simulink model "systemOffLine"  (Simulink 8.5)
settings: Solver=ode3  SolverMode=SingleTasking  StartTime=0.0  StopTime=0.1  RelTol=1e-3  AbsTol=1e-6
undefined symbols (not defined in the file or in its folder): DAB, den, elements, num
(part 1 of 5)
settings Model: Creator=PC  LastModifiedBy=PC  ExtModeTrigMode=oneshot  ExtModeArmWhenConnect=off
settings DataIOCC: LimitDataPoints=off
settings OptimizationCC: BlockReduction=off  BooleanDataType=off  ExpressionDepthLimit=128
settings DebuggingCC: SaveWithParameterizedLinksMsg=none  SignalResolutionControl=TryResolveAllWithWarning  MultiTaskDSMMsg=warning  MultiTaskCondExecSysMsg=none  FcnCallInpInsideContextMsg=EnableAllAsError  StateNameClashWarn=none
settings HardwareCC: TargetUnknown=on

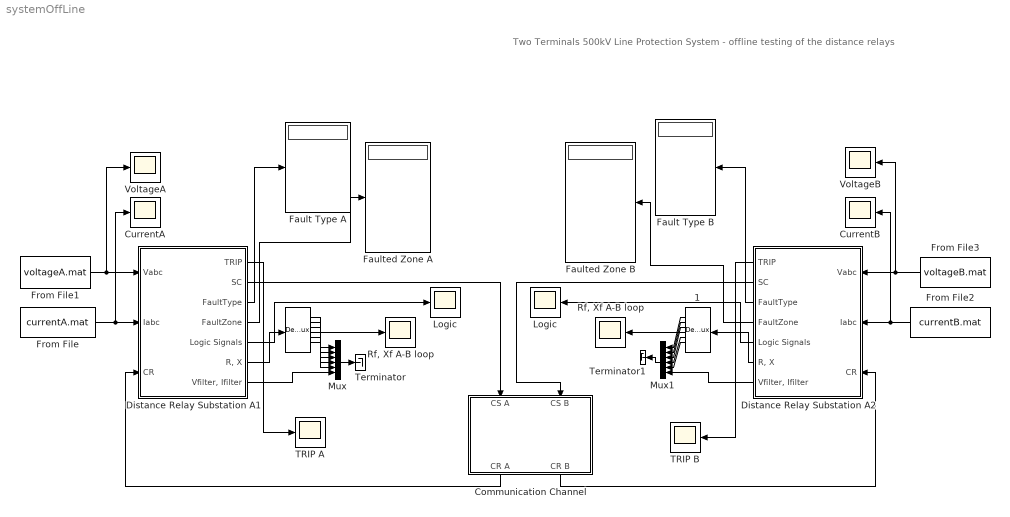
== system systemOffLine ==
  note: Two Terminals 500kV Line Protection System - offline testing of the distance relays
  "    " : Demux  Outputs=6
  "    1" : Demux  Outputs=6
  Communication Channel : Subsystem  mask(Communication channel.){Tdelay=20, failure=off, err_signal=0}
      mask prompts: Tdelay "Channel delay time [ms]:"; failure "Communication channel failure."; err_signal "Erroneous signal:"
      mask TypeOptions err_signal: 0 | 1
  CurrentA : Scope
      settings: TickLabels=on
  CurrentB : Scope
      settings: TickLabels=on
  Distance Relay Substation A1 : Subsystem  mask{ZoneImpedance=[90 115 200 250 50], ZoneTime=[0 0.33 1 0.33 0.66], k0m1=0.726, k0a1=-3.69, LineAngle=84, Zstarter=300, Tstarter=0, underV=0.8*500000/sqrt(3)*sqrt(2), PilotLogic='PUTT', fCut=180, fSampling=24*60, WindowSize=24, VoltageRange=480, CurrentRange=480}
      mask prompts: ZoneImpedance "Zone Impedances [Z1 Z2 Z3 Z4 ZR] (Ohm):"; ZoneTime "Zone Times [T1 T2 T3 T4 TR] (s):"; LineAngle "Line Angle:"; Zstarter "Starter Impedance (Ohm):"; Tstarter "Starter Time (s):"; underV "UnderVoltage Threshold (V):"; PilotLogic "Pilot Logic Scheme:"; fCut "fCut (Hz):"; fSampling "fSampling (Hz):"; WindowSize "Window Size (samples):"; VoltageRange "Voltage Range (V):"; CurrentRange "Current Range (A):"
      mask TypeOptions PilotLogic: 'BLOV+TB' | 'PUTT'
  Distance Relay Substation A2 : Subsystem  mask{ZoneImpedance=[90 115 200 250 50], ZoneTime=[0 0.33 1 0.33 0.66], k0m1=0.726, k0a1=-3.69, LineAngle=84, Zstarter=300, Tstarter=0, underV=0.8*1.05*500000/sqrt(3)*sqrt(2), PilotLogic='PUTT', fCut=180, fSampling=24*60, WindowSize=24, VoltageRange=480, CurrentRange=480}
      mask prompts: ZoneImpedance "Zone Impedances [Z1 Z2 Z3 Z4 ZR] (Ohm):"; ZoneTime "Zone Times [T1 T2 T3 T4 TR] (s):"; LineAngle "Line Angle:"; Zstarter "Starter Impedance (Ohm):"; Tstarter "Starter Time (s):"; underV "UnderVoltage Threshold (V):"; PilotLogic "Pilot Logic Scheme:"; fCut "fCut (Hz):"; fSampling "fSampling (Hz):"; WindowSize "Window Size (samples):"; VoltageRange "Voltage Range (V):"; CurrentRange "Current Range (A):"
      mask TypeOptions PilotLogic: 'BLOV+TB' | 'PUTT'
  Fault Type A : Display
  Fault Type B : Display
  Faulted Zone A : Display
  Faulted Zone B : Display
  From File : FromFile  FileName=currentA.mat  SampleTime=0
  From File1 : FromFile  FileName=voltageA.mat  SampleTime=0
  From File2 : FromFile  FileName=currentB.mat  SampleTime=0
  From File3 : FromFile  FileName=voltageB.mat  SampleTime=0
  Logic : Scope
      settings: TickLabels=on  YMin=0  YMax=1
  "Logic " : Scope
      settings: TickLabels=on  YMin=-0.5  YMax=6.5
  Mux : Mux  Inputs=6
  Mux1 : Mux  Inputs=6
  "Rf, Xf A-B loop" : Scope
      settings: TickLabels=on  YMin=-1000  YMax=2250
  "Rf, Xf A-B loop " : Scope
      settings: TickLabels=on  YMin=-150  YMax=700
  TRIP A : Scope
      settings: TickLabels=on  YMin=-1  YMax=1
  TRIP B : Scope
      settings: TickLabels=on  YMin=-1  YMax=1
  Terminator : Terminator
  Terminator1 : Terminator
  VoltageA : Scope
      settings: TickLabels=on  YMin=-450000  YMax=450000
  VoltageB : Scope
      settings: TickLabels=on  YMin=-450000  YMax=450000
  wires:
  "    1"/4 -> "Rf, Xf A-B loop "/1
  "    "/4 -> "Rf, Xf A-B loop"/1
  From File/1 -> Distance Relay Substation A1/2(Iabc), CurrentA/1
  From File1/1 -> VoltageA/1, Distance Relay Substation A1/1(Vabc)
  From File2/1 -> Distance Relay Substation A2/2(Iabc), CurrentB/1
  From File3/1 -> Distance Relay Substation A2/1(Vabc), VoltageB/1
  "    "/1 -> Mux/1
  "    "/2 -> Mux/2
  "    "/3 -> Mux/3
  "    "/5 -> Mux/4
  "    "/6 -> Mux/5
  "    1"/1 -> Mux1/1
  "    1"/2 -> Mux1/2
  "    1"/3 -> Mux1/3
  "    1"/6 -> Mux1/5
  "    1"/5 -> Mux1/4
  Mux/1 -> Terminator/1
  Mux1/1 -> Terminator1/1
  Communication Channel/1(CR A) -> Distance Relay Substation A1/3(CR)
  Distance Relay Substation A1/1("TRIP ") -> TRIP A/1
  Distance Relay Substation A1/2(SC) -> Communication Channel/1(CS A)
  Distance Relay Substation A1/3(FaultType) -> Fault Type A/1
  Distance Relay Substation A1/4(FaultZone) -> Faulted Zone A/1
  Distance Relay Substation A1/5(Logic Signals) -> Logic/1
  Distance Relay Substation A1/6("R, X") -> "    "/1
  Distance Relay Substation A1/7("Vfilter, Ifilter") -> Mux/6
  Communication Channel/2(CR B) -> Distance Relay Substation A2/3(CR)
  Distance Relay Substation A2/1("TRIP ") -> TRIP B/1
  Distance Relay Substation A2/2(SC) -> Communication Channel/2(CS B)
  Distance Relay Substation A2/3(FaultType) -> Fault Type B/1
  Distance Relay Substation A2/4(FaultZone) -> Faulted Zone B/1
  Distance Relay Substation A2/5(Logic Signals) -> "Logic "/1
  Distance Relay Substation A2/6("R, X") -> "    1"/1
  Distance Relay Substation A2/7("Vfilter, Ifilter") -> Mux1/6

== system systemOffLine/Communication Channel ==
  CS A : Inport
  CS B : Inport  Port=2
  " " : Constant  Value=failure
  "  " : Constant  Value=err_signal-1
  Switch : Switch  Threshold=0.5  SaturateOnIntegerOverflow=on  InputSameDT=on
  Switch1 : Switch  Threshold=0.5  SaturateOnIntegerOverflow=on  InputSameDT=on
  delay A->B : TransportDelay  DelayTime=Tdelay/1000  BufferSize=2048
  delay B->A : TransportDelay  DelayTime=Tdelay/1000  BufferSize=2048
  CR A : Outport  InitialOutput=0
  CR B : Outport  Port=2  InitialOutput=0
  wires:
  " "/1 -> Switch1/2, Switch/2
  delay B->A/1 -> Switch1/3
  delay A->B/1 -> Switch/3
  "  "/1 -> Switch/1, Switch1/1
  Switch1/1 -> CR B/1
  CS A/1 -> delay B->A/1
  CS B/1 -> delay A->B/1
  Switch/1 -> CR A/1

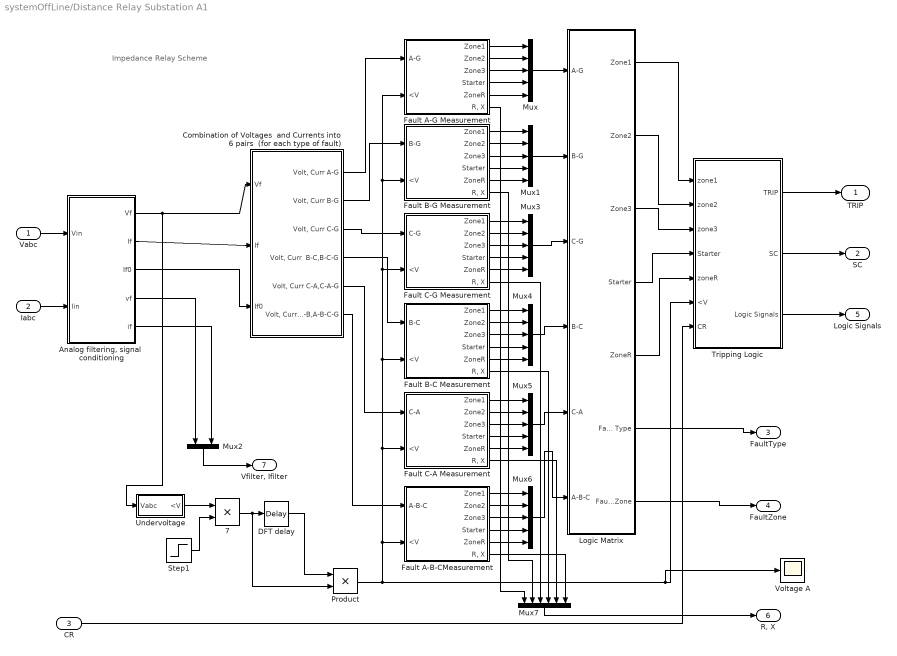
== system systemOffLine/Distance Relay Substation A1 ==
  note: Impedance Relay Scheme
  Vabc : Inport
  Iabc : Inport  Port=2
  CR : Inport  Port=3
  " 7" : Product  RndMeth=Zero
  "Analog filtering, signal  conditioning" : Subsystem
  Combination of Voltages  and Currents into 6 pairs  (for each type of fault) : Subsystem
  DFT delay : TransportDelay  DelayTime=0.017  BufferSize=30720
  Fault A-B-CMeasurement : Subsystem
  Fault A-G Measurement : Subsystem
  Fault B-C Measurement : Subsystem
  Fault B-G Measurement : Subsystem
  Fault C-A Measurement : Subsystem
  Fault C-G Measurement : Subsystem
  Logic Matrix : Subsystem
  Mux{,1,3..6} (6 alike) : Mux  Inputs=5
  Mux2 : Mux  Inputs=2
  Mux7 : Mux  Inputs=6
  Product : Product  RndMeth=Zero
  Step1 : Step  Time=0.017  SampleTime=0
  Tripping Logic : Subsystem
  Undervoltage : Subsystem
  Voltage A : Scope
      settings: TickLabels=on  YMin=-400000  YMax=400000  SaveName=ScopeData9
  "TRIP " : Outport  InitialOutput=0
  SC : Outport  Port=2  InitialOutput=0
  FaultType : Outport  Port=3  InitialOutput=0
  FaultZone : Outport  Port=4  InitialOutput=0
  Logic Signals : Outport  Port=5  InitialOutput=0
  "R, X" : Outport  Port=6  InitialOutput=0
  "Vfilter, Ifilter" : Outport  Port=7  InitialOutput=0
  wires:
  Mux2/1 -> "Vfilter, Ifilter"/1
  Product/1 -> Fault A-B-CMeasurement/2(<V), Fault C-A Measurement/2(<V), Fault B-C Measurement/2(<V), Fault C-G Measurement/2(<V), Fault B-G Measurement/2(<V), Fault A-G Measurement/2(<V), Voltage A/1, Tripping Logic/6(<V)
  Logic Matrix/6(Fault Type) -> FaultType/1
  Tripping Logic/1(TRIP) -> "TRIP "/1
  Logic Matrix/3(" Zone3") -> Tripping Logic/3(zone3)
  Logic Matrix/2(" Zone2") -> Tripping Logic/2(zone2)
  Logic Matrix/1(" Zone1") -> Tripping Logic/1(zone1)
  Mux6/1 -> Logic Matrix/6(A-B-C)
  Mux5/1 -> Logic Matrix/5(C-A)
  Mux4/1 -> Logic Matrix/4(B-C)
  Mux3/1 -> Logic Matrix/3(C-G)
  Mux1/1 -> Logic Matrix/2(B-G)
  Mux/1 -> Logic Matrix/1(A-G)
  Fault B-G Measurement/2(Zone2) -> Mux1/2
  Fault A-G Measurement/4(Starter) -> Mux/4
  Fault A-G Measurement/3(Zone3) -> Mux/3
  Fault A-G Measurement/2(Zone2) -> Mux/2
  Fault A-G Measurement/1(Zone1) -> Mux/1
  DFT delay/1 -> Product/1
  Combination of Voltages  and Currents into 6 pairs  (for each type of fault)/5("Volt, Curr C-A,C-A-G") -> Fault C-A Measurement/1(C-A)
  Combination of Voltages  and Currents into 6 pairs  (for each type of fault)/2("Volt, Curr B-G") -> Fault B-G Measurement/1(B-G)
  "Analog filtering, signal  conditioning"/3(If0) -> Combination of Voltages  and Currents into 6 pairs  (for each type of fault)/3(If0)
  "Analog filtering, signal  conditioning"/2(If) -> Combination of Voltages  and Currents into 6 pairs  (for each type of fault)/2(If)
  "Analog filtering, signal  conditioning"/5(if) -> Mux2/2
  "Analog filtering, signal  conditioning"/4(vf) -> Mux2/1
  "Analog filtering, signal  conditioning"/1(Vf) -> Undervoltage/1("Vabc  "), Combination of Voltages  and Currents into 6 pairs  (for each type of fault)/1(Vf)
  " 7"/1 -> Product/2, DFT delay/1
  Step1/1 -> " 7"/2
  Undervoltage/1(<V) -> " 7"/1
  Combination of Voltages  and Currents into 6 pairs  (for each type of fault)/1("Volt, Curr A-G") -> Fault A-G Measurement/1(A-G)
  Iabc/1 -> "Analog filtering, signal  conditioning"/2(Iin)
  Vabc/1 -> "Analog filtering, signal  conditioning"/1(Vin)
  Fault B-G Measurement/1(Zone1) -> Mux1/1
  Fault B-G Measurement/3(Zone3) -> Mux1/3
  Fault A-G Measurement/5(ZoneR) -> Mux/5
  Fault B-G Measurement/4(Starter) -> Mux1/4
  Fault B-G Measurement/5(ZoneR) -> Mux1/5
  Combination of Voltages  and Currents into 6 pairs  (for each type of fault)/3("Volt, Curr C-G") -> Fault C-G Measurement/1(C-G)
  Fault C-G Measurement/1(Zone1) -> Mux3/1
  Fault C-G Measurement/2(Zone2) -> Mux3/2
  Fault C-G Measurement/3(Zone3) -> Mux3/3
  Fault C-G Measurement/4(Starter) -> Mux3/4
  Fault C-G Measurement/5(ZoneR) -> Mux3/5
  Combination of Voltages  and Currents into 6 pairs  (for each type of fault)/4("Volt, Curr  B-C,B-C-G") -> Fault B-C Measurement/1(B-C)
  Fault B-C Measurement/1(Zone1) -> Mux4/1
  Fault B-C Measurement/2(Zone2) -> Mux4/2
  Fault B-C Measurement/3(Zone3) -> Mux4/3
  Fault B-C Measurement/4(Starter) -> Mux4/4
  Fault B-C Measurement/5(ZoneR) -> Mux4/5
  Fault C-A Measurement/1(Zone1) -> Mux5/1
  Fault C-A Measurement/2(Zone2) -> Mux5/2
  Fault C-A Measurement/3(Zone3) -> Mux5/3
  Fault C-A Measurement/4(Starter) -> Mux5/4
  Fault C-A Measurement/5(ZoneR) -> Mux5/5
  Fault A-B-CMeasurement/1(Zone1) -> Mux6/1
  Fault A-B-CMeasurement/2(Zone2) -> Mux6/2
  Fault A-B-CMeasurement/3(Zone3) -> Mux6/3
  Fault A-B-CMeasurement/4(Starter) -> Mux6/4
  Fault A-B-CMeasurement/5(ZoneR) -> Mux6/5
  Combination of Voltages  and Currents into 6 pairs  (for each type of fault)/6("Volt, Curr A-B,A-B-C-G") -> Fault A-B-CMeasurement/1(A-B-C)
  Mux7/1 -> "R, X"/1
  Fault A-B-CMeasurement/6("R, X") -> Mux7/6
  Fault C-A Measurement/6("R, X") -> Mux7/5
  Fault B-C Measurement/6("R, X") -> Mux7/4
  Fault C-G Measurement/6("R, X") -> Mux7/3
  Fault B-G Measurement/6("R, X") -> Mux7/2
  Fault A-G Measurement/6("R, X") -> Mux7/1
  Logic Matrix/7(Fault Zone) -> FaultZone/1
  Tripping Logic/2(SC) -> SC/1
  Tripping Logic/3(Logic Signals) -> Logic Signals/1
  CR/1 -> Tripping Logic/7(CR)
  Logic Matrix/4(" Starter") -> Tripping Logic/4(Starter)
  Logic Matrix/5(" ZoneR") -> Tripping Logic/5(zoneR)

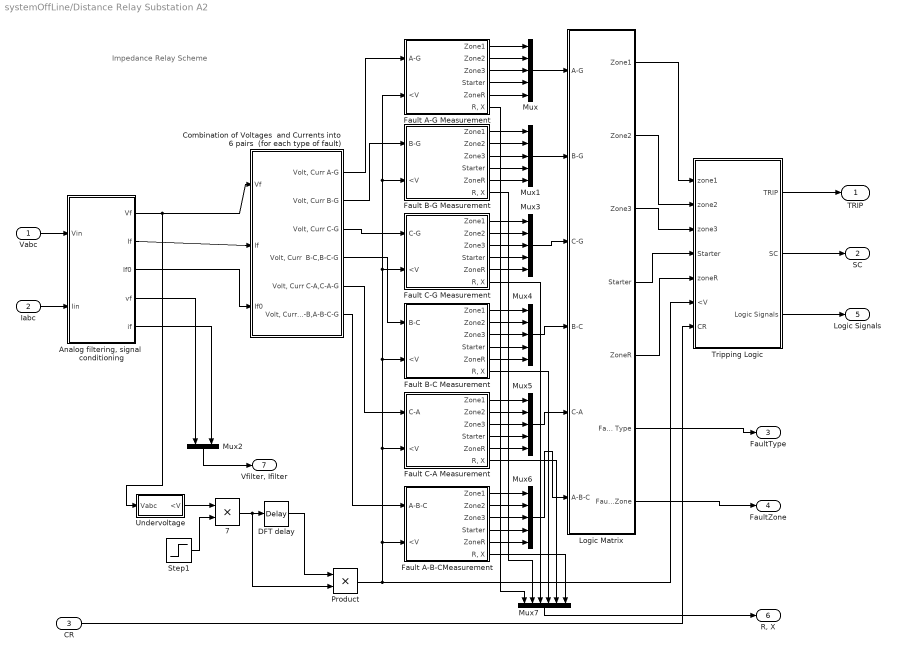
== system systemOffLine/Distance Relay Substation A2 ==
  note: Impedance Relay Scheme
  Vabc : Inport
  Iabc : Inport  Port=2
  CR : Inport  Port=3
  " 7" : Product  RndMeth=Zero
  "Analog filtering, signal  conditioning" : Subsystem
  Combination of Voltages  and Currents into 6 pairs  (for each type of fault) : Subsystem
  DFT delay : TransportDelay  DelayTime=0.017  BufferSize=30720
  Fault A-B-CMeasurement : Subsystem
  Fault A-G Measurement : Subsystem
  Fault B-C Measurement : Subsystem
  Fault B-G Measurement : Subsystem
  Fault C-A Measurement : Subsystem
  Fault C-G Measurement : Subsystem
  Logic Matrix : Subsystem
  Mux{,1,3..6} (6 alike) : Mux  Inputs=5
  Mux2 : Mux  Inputs=2
  Mux7 : Mux  Inputs=6
  Product : Product  RndMeth=Zero
  Step1 : Step  Time=0.017  SampleTime=0
  Tripping Logic : Subsystem
  Undervoltage : Subsystem
  "TRIP " : Outport  InitialOutput=0
  SC : Outport  Port=2  InitialOutput=0
  FaultType : Outport  Port=3  InitialOutput=0
  FaultZone : Outport  Port=4  InitialOutput=0
  Logic Signals : Outport  Port=5  InitialOutput=0
  "R, X" : Outport  Port=6  InitialOutput=0
  "Vfilter, Ifilter" : Outport  Port=7  InitialOutput=0
  wires:
  Mux2/1 -> "Vfilter, Ifilter"/1
  Product/1 -> Fault A-B-CMeasurement/2(<V), Fault C-A Measurement/2(<V), Fault B-C Measurement/2(<V), Fault C-G Measurement/2(<V), Fault B-G Measurement/2(<V), Fault A-G Measurement/2(<V), Tripping Logic/6(<V)
  Logic Matrix/6(Fault Type) -> FaultType/1
  Tripping Logic/1(TRIP) -> "TRIP "/1
  Logic Matrix/3(" Zone3") -> Tripping Logic/3(zone3)
  Logic Matrix/2(" Zone2") -> Tripping Logic/2(zone2)
  Logic Matrix/1(" Zone1") -> Tripping Logic/1(zone1)
  Mux6/1 -> Logic Matrix/6(A-B-C)
  Mux5/1 -> Logic Matrix/5(C-A)
  Mux4/1 -> Logic Matrix/4(B-C)
  Mux3/1 -> Logic Matrix/3(C-G)
  Mux1/1 -> Logic Matrix/2(B-G)
  Mux/1 -> Logic Matrix/1(A-G)
  Fault B-G Measurement/2(Zone2) -> Mux1/2
  Fault A-G Measurement/4(Starter) -> Mux/4
  Fault A-G Measurement/3(Zone3) -> Mux/3
  Fault A-G Measurement/2(Zone2) -> Mux/2
  Fault A-G Measurement/1(Zone1) -> Mux/1
  DFT delay/1 -> Product/1
  Combination of Voltages  and Currents into 6 pairs  (for each type of fault)/5("Volt, Curr C-A,C-A-G") -> Fault C-A Measurement/1(C-A)
  Combination of Voltages  and Currents into 6 pairs  (for each type of fault)/2("Volt, Curr B-G") -> Fault B-G Measurement/1(B-G)
  "Analog filtering, signal  conditioning"/3(If0) -> Combination of Voltages  and Currents into 6 pairs  (for each type of fault)/3(If0)
  "Analog filtering, signal  conditioning"/2(If) -> Combination of Voltages  and Currents into 6 pairs  (for each type of fault)/2(If)
  "Analog filtering, signal  conditioning"/5(if) -> Mux2/2
  "Analog filtering, signal  conditioning"/4(vf) -> Mux2/1
  "Analog filtering, signal  conditioning"/1(Vf) -> Undervoltage/1("Vabc  "), Combination of Voltages  and Currents into 6 pairs  (for each type of fault)/1(Vf)
  " 7"/1 -> Product/2, DFT delay/1
  Step1/1 -> " 7"/2
  Undervoltage/1(<V) -> " 7"/1
  Combination of Voltages  and Currents into 6 pairs  (for each type of fault)/1("Volt, Curr A-G") -> Fault A-G Measurement/1(A-G)
  Iabc/1 -> "Analog filtering, signal  conditioning"/2(Iin)
  Vabc/1 -> "Analog filtering, signal  conditioning"/1(Vin)
  Fault B-G Measurement/1(Zone1) -> Mux1/1
  Fault B-G Measurement/3(Zone3) -> Mux1/3
  Fault A-G Measurement/5(ZoneR) -> Mux/5
  Fault B-G Measurement/4(Starter) -> Mux1/4
  Fault B-G Measurement/5(ZoneR) -> Mux1/5
  Combination of Voltages  and Currents into 6 pairs  (for each type of fault)/3("Volt, Curr C-G") -> Fault C-G Measurement/1(C-G)
  Fault C-G Measurement/1(Zone1) -> Mux3/1
  Fault C-G Measurement/2(Zone2) -> Mux3/2
  Fault C-G Measurement/3(Zone3) -> Mux3/3
  Fault C-G Measurement/4(Starter) -> Mux3/4
  Fault C-G Measurement/5(ZoneR) -> Mux3/5
  Combination of Voltages  and Currents into 6 pairs  (for each type of fault)/4("Volt, Curr  B-C,B-C-G") -> Fault B-C Measurement/1(B-C)
  Fault B-C Measurement/1(Zone1) -> Mux4/1
  Fault B-C Measurement/2(Zone2) -> Mux4/2
  Fault B-C Measurement/3(Zone3) -> Mux4/3
  Fault B-C Measurement/4(Starter) -> Mux4/4
  Fault B-C Measurement/5(ZoneR) -> Mux4/5
  Fault C-A Measurement/1(Zone1) -> Mux5/1
  Fault C-A Measurement/2(Zone2) -> Mux5/2
  Fault C-A Measurement/3(Zone3) -> Mux5/3
  Fault C-A Measurement/4(Starter) -> Mux5/4
  Fault C-A Measurement/5(ZoneR) -> Mux5/5
  Fault A-B-CMeasurement/1(Zone1) -> Mux6/1
  Fault A-B-CMeasurement/2(Zone2) -> Mux6/2
  Fault A-B-CMeasurement/3(Zone3) -> Mux6/3
  Fault A-B-CMeasurement/4(Starter) -> Mux6/4
  Fault A-B-CMeasurement/5(ZoneR) -> Mux6/5
  Combination of Voltages  and Currents into 6 pairs  (for each type of fault)/6("Volt, Curr A-B,A-B-C-G") -> Fault A-B-CMeasurement/1(A-B-C)
  Mux7/1 -> "R, X"/1
  Fault A-B-CMeasurement/6("R, X") -> Mux7/6
  Fault C-A Measurement/6("R, X") -> Mux7/5
  Fault B-C Measurement/6("R, X") -> Mux7/4
  Fault C-G Measurement/6("R, X") -> Mux7/3
  Fault B-G Measurement/6("R, X") -> Mux7/2
  Fault A-G Measurement/6("R, X") -> Mux7/1
  Logic Matrix/7(Fault Zone) -> FaultZone/1
  Tripping Logic/2(SC) -> SC/1
  Tripping Logic/3(Logic Signals) -> Logic Signals/1
  CR/1 -> Tripping Logic/7(CR)
  Logic Matrix/4(" Starter") -> Tripping Logic/4(Starter)
  Logic Matrix/5(" ZoneR") -> Tripping Logic/5(zoneR)

== system systemOffLine/Distance Relay Substation A1/Analog filtering, signal  conditioning ==
  note: Acquisition Block- analog filtering,
      | signal conditioning, sampling.
  Vin : Inport
  Iin : Inport  Port=2
  CURRENTS : Subsystem
  Mux{1..4} (4 alike) : Mux  Inputs=3
  VOLTAGES : Subsystem
  Vf : Outport  InitialOutput=0
  If : Outport  Port=2  InitialOutput=0
  If0 : Outport  Port=3  InitialOutput=0
  vf : Outport  Port=4  InitialOutput=0
  if : Outport  Port=5  InitialOutput=0
  wires:
  CURRENTS/4(k0I0f) -> If0/1
  Mux4/1 -> if/1
  Mux3/1 -> If/1
  CURRENTS/7(icf) -> Mux4/3
  CURRENTS/6(ibf) -> Mux4/2
  CURRENTS/5(iaf) -> Mux4/1
  CURRENTS/3(ICf) -> Mux3/3
  CURRENTS/2(IBf) -> Mux3/2
  CURRENTS/1(IAf) -> Mux3/1
  Iin/1 -> CURRENTS/1(Iabc)
  Mux2/1 -> vf/1
  VOLTAGES/6(vcf) -> Mux2/3
  VOLTAGES/5(vbf) -> Mux2/2
  VOLTAGES/4(vaf) -> Mux2/1
  VOLTAGES/3(VCf) -> Mux1/3
  VOLTAGES/2(VBf) -> Mux1/2
  VOLTAGES/1(VAf) -> Mux1/1
  Vin/1 -> VOLTAGES/1(Vabc)
  Mux1/1 -> Vf/1

== system systemOffLine/Distance Relay Substation A1/Combination of Voltages  and Currents into 6 pairs  (for each type of fault) ==
  note: Voltage and current combination block
  Vf : Inport
  If : Inport  Port=2
  If0 : Inport  Port=3
  "Currents Ia, Ib, Ic, kIo" : Demux  Outputs=3
  Ia+kIo : Sum  SaturateOnIntegerOverflow=on  InputSameDT=on  OutDataTypeStr=Inherit: Same as first input
  Ia-Ib : Sum  Inputs=+-  SaturateOnIntegerOverflow=on  InputSameDT=on  OutDataTypeStr=Inherit: Same as first input
  Ib+kIo : Sum  SaturateOnIntegerOverflow=on  InputSameDT=on  OutDataTypeStr=Inherit: Same as first input
  Ib-Ic : Sum  Inputs=+-  SaturateOnIntegerOverflow=on  InputSameDT=on  OutDataTypeStr=Inherit: Same as first input
  Ic+kIo : Sum  SaturateOnIntegerOverflow=on  InputSameDT=on  OutDataTypeStr=Inherit: Same as first input
  Ic-Ia : Sum  Inputs=+-  SaturateOnIntegerOverflow=on  InputSameDT=on  OutDataTypeStr=Inherit: Same as first input
  Mux{10..15} (6 alike) : Mux  Inputs=2
  Va-Vb : Sum  Inputs=+-  SaturateOnIntegerOverflow=on  InputSameDT=on  OutDataTypeStr=Inherit: Same as first input
  Vb-Vc : Sum  Inputs=+-  SaturateOnIntegerOverflow=on  InputSameDT=on  OutDataTypeStr=Inherit: Same as first input
  Vc-Va : Sum  Inputs=+-  SaturateOnIntegerOverflow=on  InputSameDT=on  OutDataTypeStr=Inherit: Same as first input
  "Voltages Va,Vb, Vc" : Demux  Outputs=3
  "Volt, Curr A-G" : Outport  InitialOutput=0
  "Volt, Curr B-G" : Outport  Port=2  InitialOutput=0
  "Volt, Curr C-G" : Outport  Port=3  InitialOutput=0
  "Volt, Curr  B-C,B-C-G" : Outport  Port=4  InitialOutput=0
  "Volt, Curr C-A,C-A-G" : Outport  Port=5  InitialOutput=0
  "Volt, Curr A-B,A-B-C-G" : Outport  Port=6  InitialOutput=0
  wires:
  If0/1 -> Ib+kIo/2, Ia+kIo/2, Ic+kIo/2
  Mux13/1 -> "Volt, Curr  B-C,B-C-G"/1
  Vb-Vc/1 -> Mux13/1
  Ib-Ic/1 -> Mux13/2
  Mux12/1 -> "Volt, Curr C-G"/1
  Ic+kIo/1 -> Mux12/2
  If/1 -> "Currents Ia, Ib, Ic, kIo"/1
  "Voltages Va,Vb, Vc"/3 -> Vc-Va/1, Vb-Vc/2, Mux12/1
  "Voltages Va,Vb, Vc"/2 -> Vb-Vc/1, Mux11/1, Va-Vb/2
  "Voltages Va,Vb, Vc"/1 -> Va-Vb/1, Mux10/1, Vc-Va/2
  Vf/1 -> "Voltages Va,Vb, Vc"/1
  Mux15/1 -> "Volt, Curr A-B,A-B-C-G"/1
  Mux14/1 -> "Volt, Curr C-A,C-A-G"/1
  Vc-Va/1 -> Mux14/1
  Mux11/1 -> "Volt, Curr B-G"/1
  Mux10/1 -> "Volt, Curr A-G"/1
  Ia+kIo/1 -> Mux10/2
  Ib+kIo/1 -> Mux11/2
  Ic-Ia/1 -> Mux14/2
  Va-Vb/1 -> Mux15/1
  Ia-Ib/1 -> Mux15/2
  "Currents Ia, Ib, Ic, kIo"/2 -> Ia-Ib/2, Ib-Ic/1, Ib+kIo/1
  "Currents Ia, Ib, Ic, kIo"/3 -> Ic-Ia/1, Ib-Ic/2, Ic+kIo/1
  "Currents Ia, Ib, Ic, kIo"/1 -> Ia-Ib/1, Ic-Ia/2, Ia+kIo/1

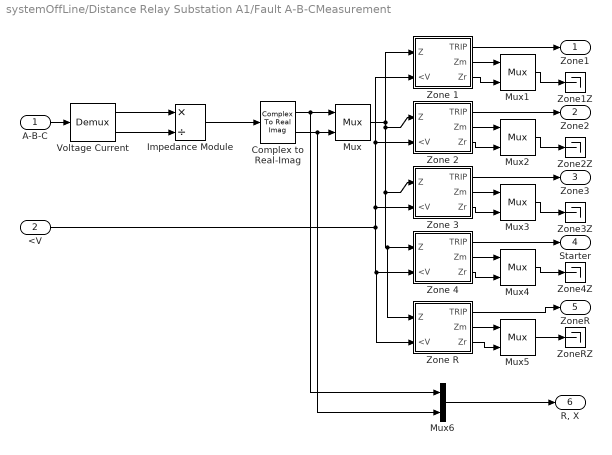
== system systemOffLine/Distance Relay Substation A1/Fault A-B-CMeasurement ==
  A-B-C : Inport
  <V : Inport  Port=2
  Complex to Real-Imag : ComplexToRealImag
  Impedance Module : Product  Inputs=*/  SaturateOnIntegerOverflow=on  RndMeth=Zero  InputSameDT=on  OutDataTypeStr=Inherit: Same as first input
  Mux{,1..6} (7 alike) : Mux  Inputs=2
  Voltage Current : Demux  Outputs=2
  Zone 1 : Subsystem  mask(Zone){Xr=ZoneImpedance(1)*sin(LineAngle*pi/180), Rr=ZoneImpedance(1)*cos(LineAngle*pi/180), Td=ZoneTime(1)}
      mask prompts: Xr "Reactance reach [ohm]"; Rr "Resistance reach [ohm]"; Td "Time delay [s]"
  Zone 2 : Subsystem  mask(Zone){Xr=ZoneImpedance(2)*sin(LineAngle*pi/180), Rr=ZoneImpedance(2)*cos(LineAngle*pi/180), Td=ZoneTime(2)}
      mask prompts: Xr "Reactance reach [ohm]"; Rr "Resistance reach [ohm]"; Td "Time delay [s]"
  Zone 3 : Subsystem  mask(Zone){Xr=ZoneImpedance(3)*sin(LineAngle*pi/180), Rr=ZoneImpedance(3)*cos(LineAngle*pi/180), Td=ZoneTime(3)}
      mask prompts: Xr "Reactance reach [ohm]"; Rr "Resistance reach [ohm]"; Td "Time delay [s]"
  Zone 4 : Subsystem  mask(Zone){Xr=ZoneImpedance(4)*sin(LineAngle*pi/180), Rr=ZoneImpedance(4)*cos(LineAngle*pi/180), Td=ZoneTime(4)}
      mask prompts: Xr "Reactance reach [ohm]"; Rr "Resistance reach [ohm]"; Td "Time delay [s]"
  Zone R : Subsystem  mask(Zone){Xr=ZoneImpedance(5)*sin(LineAngle*pi/180), Rr=ZoneImpedance(5)*cos(LineAngle*pi/180), Td=ZoneTime(5)}
      mask prompts: Xr "Reactance reach [ohm]"; Rr "Resistance reach [ohm]"; Td "Time delay [s]"
  Zone1Z : Terminator
  Zone2Z : Terminator
  Zone3Z : Terminator
  Zone4Z : Terminator
  ZoneRZ : Terminator
  Zone1 : Outport  InitialOutput=0
  Zone2 : Outport  Port=2  InitialOutput=0
  Zone3 : Outport  Port=3  InitialOutput=0
  Starter : Outport  Port=4  InitialOutput=0
  ZoneR : Outport  Port=5  InitialOutput=0
  "R, X" : Outport  Port=6  InitialOutput=0
  wires:
  Voltage Current/2 -> Impedance Module/2
  Voltage Current/1 -> Impedance Module/1
  Impedance Module/1 -> Complex to Real-Imag/1
  Mux4/1 -> Zone4Z/1
  Mux3/1 -> Zone3Z/1
  Mux2/1 -> Zone2Z/1
  Mux1/1 -> Zone1Z/1
  <V/1 -> Zone R/2(<V), Zone 4/2(<V), Zone 3/2(<V), Zone 2/2(<V), Zone 1/2(<V)
  Complex to Real-Imag/2 -> Mux6/2, Mux/2
  Complex to Real-Imag/1 -> Mux6/1, Mux/1
  Zone 4/1(TRIP) -> Starter/1
  Zone 3/1(TRIP) -> Zone3/1
  Zone 2/1(TRIP) -> Zone2/1
  Zone 4/3(Zr) -> Mux4/2
  Zone 4/2(Zm) -> Mux4/1
  Zone 3/3(Zr) -> Mux3/2
  Zone 3/2(Zm) -> Mux3/1
  Zone 2/3(Zr) -> Mux2/2
  Zone 2/2(Zm) -> Mux2/1
  Zone 1/3(Zr) -> Mux1/2
  Zone 1/2(Zm) -> Mux1/1
  Zone 1/1(TRIP) -> Zone1/1
  Mux/1 -> Zone 2/1(Z), Zone R/1(Z), Zone 4/1(Z), Zone 3/1(Z), Zone 1/1(Z)
  A-B-C/1 -> Voltage Current/1
  Zone R/2(Zm) -> Mux5/1
  Zone R/3(Zr) -> Mux5/2
  Mux5/1 -> ZoneRZ/1
  Zone R/1(TRIP) -> ZoneR/1
  Mux6/1 -> "R, X"/1

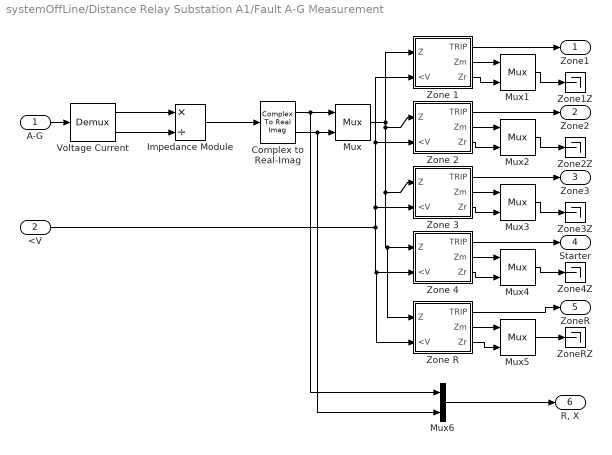
== system systemOffLine/Distance Relay Substation A1/Fault A-G Measurement ==
  A-G : Inport
  <V : Inport  Port=2
  Complex to Real-Imag : ComplexToRealImag
  Impedance Module : Product  Inputs=*/  SaturateOnIntegerOverflow=on  RndMeth=Zero  InputSameDT=on  OutDataTypeStr=Inherit: Same as first input
  Mux{,1..6} (7 alike) : Mux  Inputs=2
  Voltage Current : Demux  Outputs=2
  Zone 1 : Subsystem  mask(Zone){Xr=ZoneImpedance(1)*sin(LineAngle*pi/180), Rr=ZoneImpedance(1)*cos(LineAngle*pi/180), Td=ZoneTime(1)}
      mask prompts: Xr "Reactance reach [ohm]"; Rr "Resistance reach [ohm]"; Td "Time delay [s]"
  Zone 2 : Subsystem  mask(Zone){Xr=ZoneImpedance(2)*sin(LineAngle*pi/180), Rr=ZoneImpedance(2)*cos(LineAngle*pi/180), Td=ZoneTime(2)}
      mask prompts: Xr "Reactance reach [ohm]"; Rr "Resistance reach [ohm]"; Td "Time delay [s]"
  Zone 3 : Subsystem  mask(Zone){Xr=ZoneImpedance(3)*sin(LineAngle*pi/180), Rr=ZoneImpedance(3)*cos(LineAngle*pi/180), Td=ZoneTime(3)}
      mask prompts: Xr "Reactance reach [ohm]"; Rr "Resistance reach [ohm]"; Td "Time delay [s]"
  Zone 4 : Subsystem  mask(Zone){Xr=ZoneImpedance(4)*sin(LineAngle*pi/180), Rr=ZoneImpedance(4)*cos(LineAngle*pi/180), Td=ZoneTime(4)}
      mask prompts: Xr "Reactance reach [ohm]"; Rr "Resistance reach [ohm]"; Td "Time delay [s]"
  Zone R : Subsystem  mask(Zone){Xr=ZoneImpedance(5)*sin(LineAngle*pi/180), Rr=ZoneImpedance(5)*cos(LineAngle*pi/180), Td=ZoneTime(5)}
      mask prompts: Xr "Reactance reach [ohm]"; Rr "Resistance reach [ohm]"; Td "Time delay [s]"
  Zone1Z : Terminator
  Zone2Z : Terminator
  Zone3Z : Terminator
  Zone4Z : Terminator
  ZoneRZ : Terminator
  Zone1 : Outport  InitialOutput=0
  Zone2 : Outport  Port=2  InitialOutput=0
  Zone3 : Outport  Port=3  InitialOutput=0
  Starter : Outport  Port=4  InitialOutput=0
  ZoneR : Outport  Port=5  InitialOutput=0
  "R, X" : Outport  Port=6  InitialOutput=0
  wires:
  Voltage Current/2 -> Impedance Module/2
  Voltage Current/1 -> Impedance Module/1
  Impedance Module/1 -> Complex to Real-Imag/1
  Mux4/1 -> Zone4Z/1
  Mux3/1 -> Zone3Z/1
  Mux2/1 -> Zone2Z/1
  Mux1/1 -> Zone1Z/1
  <V/1 -> Zone R/2(<V), Zone 4/2(<V), Zone 3/2(<V), Zone 2/2(<V), Zone 1/2(<V)
  Complex to Real-Imag/2 -> Mux6/2, Mux/2
  Complex to Real-Imag/1 -> Mux6/1, Mux/1
  Zone 4/1(TRIP) -> Starter/1
  Zone 3/1(TRIP) -> Zone3/1
  Zone 2/1(TRIP) -> Zone2/1
  Zone 4/3(Zr) -> Mux4/2
  Zone 4/2(Zm) -> Mux4/1
  Zone 3/3(Zr) -> Mux3/2
  Zone 3/2(Zm) -> Mux3/1
  Zone 2/3(Zr) -> Mux2/2
  Zone 2/2(Zm) -> Mux2/1
  Zone 1/3(Zr) -> Mux1/2
  Zone 1/2(Zm) -> Mux1/1
  Zone 1/1(TRIP) -> Zone1/1
  Mux/1 -> Zone 2/1(Z), Zone R/1(Z), Zone 4/1(Z), Zone 3/1(Z), Zone 1/1(Z)
  A-G/1 -> Voltage Current/1
  Zone R/2(Zm) -> Mux5/1
  Zone R/3(Zr) -> Mux5/2
  Mux5/1 -> ZoneRZ/1
  Zone R/1(TRIP) -> ZoneR/1
  Mux6/1 -> "R, X"/1

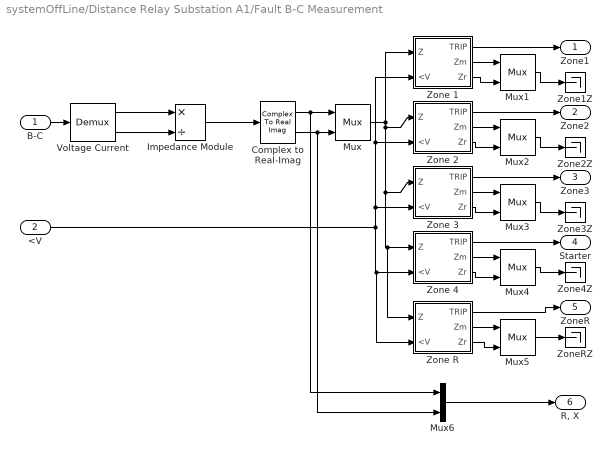
== system systemOffLine/Distance Relay Substation A1/Fault B-C Measurement ==
  B-C : Inport
  <V : Inport  Port=2
  Complex to Real-Imag : ComplexToRealImag
  Impedance Module : Product  Inputs=*/  SaturateOnIntegerOverflow=on  RndMeth=Zero  InputSameDT=on  OutDataTypeStr=Inherit: Same as first input
  Mux{,1..6} (7 alike) : Mux  Inputs=2
  Voltage Current : Demux  Outputs=2
  Zone 1 : Subsystem  mask(Zone){Xr=ZoneImpedance(1)*sin(LineAngle*pi/180), Rr=ZoneImpedance(1)*cos(LineAngle*pi/180), Td=ZoneTime(1)}
      mask prompts: Xr "Reactance reach [ohm]"; Rr "Resistance reach [ohm]"; Td "Time delay [s]"
  Zone 2 : Subsystem  mask(Zone){Xr=ZoneImpedance(2)*sin(LineAngle*pi/180), Rr=ZoneImpedance(2)*cos(LineAngle*pi/180), Td=ZoneTime(2)}
      mask prompts: Xr "Reactance reach [ohm]"; Rr "Resistance reach [ohm]"; Td "Time delay [s]"
  Zone 3 : Subsystem  mask(Zone){Xr=ZoneImpedance(3)*sin(LineAngle*pi/180), Rr=ZoneImpedance(3)*cos(LineAngle*pi/180), Td=ZoneTime(3)}
      mask prompts: Xr "Reactance reach [ohm]"; Rr "Resistance reach [ohm]"; Td "Time delay [s]"
  Zone 4 : Subsystem  mask(Zone){Xr=ZoneImpedance(4)*sin(LineAngle*pi/180), Rr=ZoneImpedance(4)*cos(LineAngle*pi/180), Td=ZoneTime(4)}
      mask prompts: Xr "Reactance reach [ohm]"; Rr "Resistance reach [ohm]"; Td "Time delay [s]"
  Zone R : Subsystem  mask(Zone){Xr=ZoneImpedance(5)*sin(LineAngle*pi/180), Rr=ZoneImpedance(5)*cos(LineAngle*pi/180), Td=ZoneTime(5)}
      mask prompts: Xr "Reactance reach [ohm]"; Rr "Resistance reach [ohm]"; Td "Time delay [s]"
  Zone1Z : Terminator
  Zone2Z : Terminator
  Zone3Z : Terminator
  Zone4Z : Terminator
  ZoneRZ : Terminator
  Zone1 : Outport  InitialOutput=0
  Zone2 : Outport  Port=2  InitialOutput=0
  Zone3 : Outport  Port=3  InitialOutput=0
  Starter : Outport  Port=4  InitialOutput=0
  ZoneR : Outport  Port=5  InitialOutput=0
  "R, X" : Outport  Port=6  InitialOutput=0
  wires:
  Voltage Current/2 -> Impedance Module/2
  Voltage Current/1 -> Impedance Module/1
  Impedance Module/1 -> Complex to Real-Imag/1
  Mux4/1 -> Zone4Z/1
  Mux3/1 -> Zone3Z/1
  Mux2/1 -> Zone2Z/1
  Mux1/1 -> Zone1Z/1
  <V/1 -> Zone R/2(<V), Zone 4/2(<V), Zone 3/2(<V), Zone 2/2(<V), Zone 1/2(<V)
  Complex to Real-Imag/2 -> Mux6/2, Mux/2
  Complex to Real-Imag/1 -> Mux6/1, Mux/1
  Zone 4/1(TRIP) -> Starter/1
  Zone 3/1(TRIP) -> Zone3/1
  Zone 2/1(TRIP) -> Zone2/1
  Zone 4/3(Zr) -> Mux4/2
  Zone 4/2(Zm) -> Mux4/1
  Zone 3/3(Zr) -> Mux3/2
  Zone 3/2(Zm) -> Mux3/1
  Zone 2/3(Zr) -> Mux2/2
  Zone 2/2(Zm) -> Mux2/1
  Zone 1/3(Zr) -> Mux1/2
  Zone 1/2(Zm) -> Mux1/1
  Zone 1/1(TRIP) -> Zone1/1
  Mux/1 -> Zone 2/1(Z), Zone R/1(Z), Zone 4/1(Z), Zone 3/1(Z), Zone 1/1(Z)
  B-C/1 -> Voltage Current/1
  Zone R/2(Zm) -> Mux5/1
  Zone R/3(Zr) -> Mux5/2
  Mux5/1 -> ZoneRZ/1
  Zone R/1(TRIP) -> ZoneR/1
  Mux6/1 -> "R, X"/1

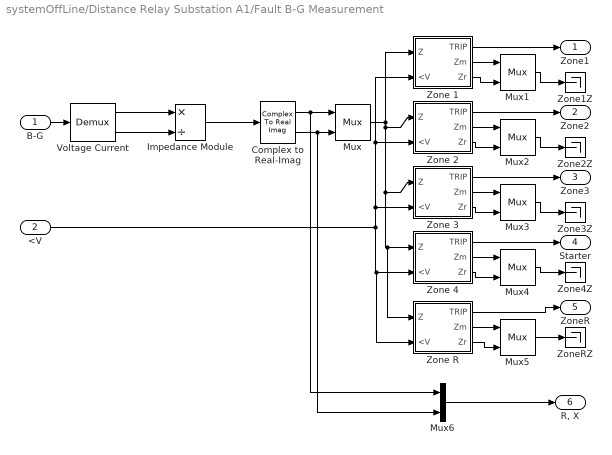
== system systemOffLine/Distance Relay Substation A1/Fault B-G Measurement ==
  B-G : Inport
  <V : Inport  Port=2
  Complex to Real-Imag : ComplexToRealImag
  Impedance Module : Product  Inputs=*/  SaturateOnIntegerOverflow=on  RndMeth=Zero  InputSameDT=on  OutDataTypeStr=Inherit: Same as first input
  Mux{,1..6} (7 alike) : Mux  Inputs=2
  Voltage Current : Demux  Outputs=2
  Zone 1 : Subsystem  mask(Zone){Xr=ZoneImpedance(1)*sin(LineAngle*pi/180), Rr=ZoneImpedance(1)*cos(LineAngle*pi/180), Td=ZoneTime(1)}
      mask prompts: Xr "Reactance reach [ohm]"; Rr "Resistance reach [ohm]"; Td "Time delay [s]"
  Zone 2 : Subsystem  mask(Zone){Xr=ZoneImpedance(2)*sin(LineAngle*pi/180), Rr=ZoneImpedance(2)*cos(LineAngle*pi/180), Td=ZoneTime(2)}
      mask prompts: Xr "Reactance reach [ohm]"; Rr "Resistance reach [ohm]"; Td "Time delay [s]"
  Zone 3 : Subsystem  mask(Zone){Xr=ZoneImpedance(3)*sin(LineAngle*pi/180), Rr=ZoneImpedance(3)*cos(LineAngle*pi/180), Td=ZoneTime(3)}
      mask prompts: Xr "Reactance reach [ohm]"; Rr "Resistance reach [ohm]"; Td "Time delay [s]"
  Zone 4 : Subsystem  mask(Zone){Xr=ZoneImpedance(4)*sin(LineAngle*pi/180), Rr=ZoneImpedance(4)*cos(LineAngle*pi/180), Td=ZoneTime(4)}
      mask prompts: Xr "Reactance reach [ohm]"; Rr "Resistance reach [ohm]"; Td "Time delay [s]"
  Zone R : Subsystem  mask(Zone){Xr=ZoneImpedance(5)*sin(LineAngle*pi/180), Rr=ZoneImpedance(5)*cos(LineAngle*pi/180), Td=ZoneTime(5)}
      mask prompts: Xr "Reactance reach [ohm]"; Rr "Resistance reach [ohm]"; Td "Time delay [s]"
  Zone1Z : Terminator
  Zone2Z : Terminator
  Zone3Z : Terminator
  Zone4Z : Terminator
  ZoneRZ : Terminator
  Zone1 : Outport  InitialOutput=0
  Zone2 : Outport  Port=2  InitialOutput=0
  Zone3 : Outport  Port=3  InitialOutput=0
  Starter : Outport  Port=4  InitialOutput=0
  ZoneR : Outport  Port=5  InitialOutput=0
  "R, X" : Outport  Port=6  InitialOutput=0
  wires:
  Voltage Current/2 -> Impedance Module/2
  Voltage Current/1 -> Impedance Module/1
  Impedance Module/1 -> Complex to Real-Imag/1
  Mux4/1 -> Zone4Z/1
  Mux3/1 -> Zone3Z/1
  Mux2/1 -> Zone2Z/1
  Mux1/1 -> Zone1Z/1
  <V/1 -> Zone R/2(<V), Zone 4/2(<V), Zone 3/2(<V), Zone 2/2(<V), Zone 1/2(<V)
  Complex to Real-Imag/2 -> Mux6/2, Mux/2
  Complex to Real-Imag/1 -> Mux6/1, Mux/1
  Zone 4/1(TRIP) -> Starter/1
  Zone 3/1(TRIP) -> Zone3/1
  Zone 2/1(TRIP) -> Zone2/1
  Zone 4/3(Zr) -> Mux4/2
  Zone 4/2(Zm) -> Mux4/1
  Zone 3/3(Zr) -> Mux3/2
  Zone 3/2(Zm) -> Mux3/1
  Zone 2/3(Zr) -> Mux2/2
  Zone 2/2(Zm) -> Mux2/1
  Zone 1/3(Zr) -> Mux1/2
  Zone 1/2(Zm) -> Mux1/1
  Zone 1/1(TRIP) -> Zone1/1
  Mux/1 -> Zone 2/1(Z), Zone R/1(Z), Zone 4/1(Z), Zone 3/1(Z), Zone 1/1(Z)
  B-G/1 -> Voltage Current/1
  Zone R/2(Zm) -> Mux5/1
  Zone R/3(Zr) -> Mux5/2
  Mux5/1 -> ZoneRZ/1
  Zone R/1(TRIP) -> ZoneR/1
  Mux6/1 -> "R, X"/1

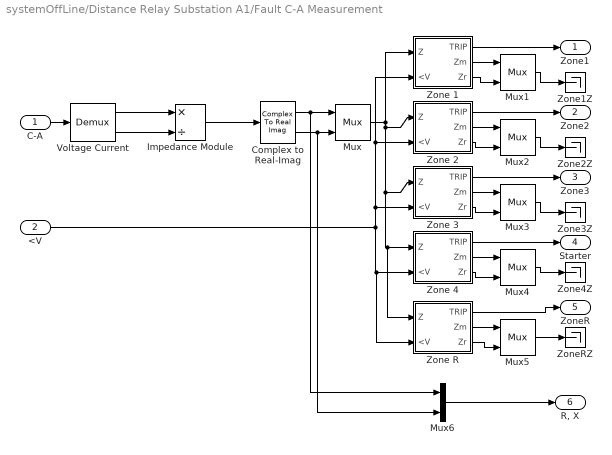
== system systemOffLine/Distance Relay Substation A1/Fault C-A Measurement ==
  C-A : Inport
  <V : Inport  Port=2
  Complex to Real-Imag : ComplexToRealImag
  Impedance Module : Product  Inputs=*/  SaturateOnIntegerOverflow=on  RndMeth=Zero  InputSameDT=on  OutDataTypeStr=Inherit: Same as first input
  Mux{,1..6} (7 alike) : Mux  Inputs=2
  Voltage Current : Demux  Outputs=2
  Zone 1 : Subsystem  mask(Zone){Xr=ZoneImpedance(1)*sin(LineAngle*pi/180), Rr=ZoneImpedance(1)*cos(LineAngle*pi/180), Td=ZoneTime(1)}
      mask prompts: Xr "Reactance reach [ohm]"; Rr "Resistance reach [ohm]"; Td "Time delay [s]"
  Zone 2 : Subsystem  mask(Zone){Xr=ZoneImpedance(2)*sin(LineAngle*pi/180), Rr=ZoneImpedance(2)*cos(LineAngle*pi/180), Td=ZoneTime(2)}
      mask prompts: Xr "Reactance reach [ohm]"; Rr "Resistance reach [ohm]"; Td "Time delay [s]"
  Zone 3 : Subsystem  mask(Zone){Xr=ZoneImpedance(3)*sin(LineAngle*pi/180), Rr=ZoneImpedance(3)*cos(LineAngle*pi/180), Td=ZoneTime(3)}
      mask prompts: Xr "Reactance reach [ohm]"; Rr "Resistance reach [ohm]"; Td "Time delay [s]"
  Zone 4 : Subsystem  mask(Zone){Xr=ZoneImpedance(4)*sin(LineAngle*pi/180), Rr=ZoneImpedance(4)*cos(LineAngle*pi/180), Td=ZoneTime(4)}
      mask prompts: Xr "Reactance reach [ohm]"; Rr "Resistance reach [ohm]"; Td "Time delay [s]"
  Zone R : Subsystem  mask(Zone){Xr=ZoneImpedance(5)*sin(LineAngle*pi/180), Rr=ZoneImpedance(5)*cos(LineAngle*pi/180), Td=ZoneTime(5)}
      mask prompts: Xr "Reactance reach [ohm]"; Rr "Resistance reach [ohm]"; Td "Time delay [s]"
  Zone1Z : Terminator
  Zone2Z : Terminator
  Zone3Z : Terminator
  Zone4Z : Terminator
  ZoneRZ : Terminator
  Zone1 : Outport  InitialOutput=0
  Zone2 : Outport  Port=2  InitialOutput=0
  Zone3 : Outport  Port=3  InitialOutput=0
  Starter : Outport  Port=4  InitialOutput=0
  ZoneR : Outport  Port=5  InitialOutput=0
  "R, X" : Outport  Port=6  InitialOutput=0
  wires:
  Voltage Current/2 -> Impedance Module/2
  Voltage Current/1 -> Impedance Module/1
  Impedance Module/1 -> Complex to Real-Imag/1
  Mux4/1 -> Zone4Z/1
  Mux3/1 -> Zone3Z/1
  Mux2/1 -> Zone2Z/1
  Mux1/1 -> Zone1Z/1
  <V/1 -> Zone R/2(<V), Zone 4/2(<V), Zone 3/2(<V), Zone 2/2(<V), Zone 1/2(<V)
  Complex to Real-Imag/2 -> Mux6/2, Mux/2
  Complex to Real-Imag/1 -> Mux6/1, Mux/1
  Zone 4/1(TRIP) -> Starter/1
  Zone 3/1(TRIP) -> Zone3/1
  Zone 2/1(TRIP) -> Zone2/1
  Zone 4/3(Zr) -> Mux4/2
  Zone 4/2(Zm) -> Mux4/1
  Zone 3/3(Zr) -> Mux3/2
  Zone 3/2(Zm) -> Mux3/1
  Zone 2/3(Zr) -> Mux2/2
  Zone 2/2(Zm) -> Mux2/1
  Zone 1/3(Zr) -> Mux1/2
  Zone 1/2(Zm) -> Mux1/1
  Zone 1/1(TRIP) -> Zone1/1
  Mux/1 -> Zone 2/1(Z), Zone R/1(Z), Zone 4/1(Z), Zone 3/1(Z), Zone 1/1(Z)
  C-A/1 -> Voltage Current/1
  Zone R/2(Zm) -> Mux5/1
  Zone R/3(Zr) -> Mux5/2
  Mux5/1 -> ZoneRZ/1
  Zone R/1(TRIP) -> ZoneR/1
  Mux6/1 -> "R, X"/1

== system systemOffLine/Distance Relay Substation A1/Fault C-G Measurement ==
  C-G : Inport
  <V : Inport  Port=2
  Complex to Real-Imag : ComplexToRealImag
  Impedance Module : Product  Inputs=*/  SaturateOnIntegerOverflow=on  RndMeth=Zero  InputSameDT=on  OutDataTypeStr=Inherit: Same as first input
  Mux{,1..6} (7 alike) : Mux  Inputs=2
  Voltage Current : Demux  Outputs=2
  Zone 1 : Subsystem  mask(Zone){Xr=ZoneImpedance(1)*sin(LineAngle*pi/180), Rr=ZoneImpedance(1)*cos(LineAngle*pi/180), Td=ZoneTime(1)}
      mask prompts: Xr "Reactance reach [ohm]"; Rr "Resistance reach [ohm]"; Td "Time delay [s]"
  Zone 2 : Subsystem  mask(Zone){Xr=ZoneImpedance(2)*sin(LineAngle*pi/180), Rr=ZoneImpedance(2)*cos(LineAngle*pi/180), Td=ZoneTime(2)}
      mask prompts: Xr "Reactance reach [ohm]"; Rr "Resistance reach [ohm]"; Td "Time delay [s]"
  Zone 3 : Subsystem  mask(Zone){Xr=ZoneImpedance(3)*sin(LineAngle*pi/180), Rr=ZoneImpedance(3)*cos(LineAngle*pi/180), Td=ZoneTime(3)}
      mask prompts: Xr "Reactance reach [ohm]"; Rr "Resistance reach [ohm]"; Td "Time delay [s]"
  Zone 4 : Subsystem  mask(Zone){Xr=ZoneImpedance(4)*sin(LineAngle*pi/180), Rr=ZoneImpedance(4)*cos(LineAngle*pi/180), Td=ZoneTime(4)}
      mask prompts: Xr "Reactance reach [ohm]"; Rr "Resistance reach [ohm]"; Td "Time delay [s]"
  Zone R : Subsystem  mask(Zone){Xr=ZoneImpedance(5)*sin(LineAngle*pi/180), Rr=ZoneImpedance(5)*cos(LineAngle*pi/180), Td=ZoneTime(5)}
      mask prompts: Xr "Reactance reach [ohm]"; Rr "Resistance reach [ohm]"; Td "Time delay [s]"
  Zone1Z : Terminator
  Zone2Z : Terminator
  Zone3Z : Terminator
  Zone4Z : Terminator
  ZoneRZ : Terminator
  Zone1 : Outport  InitialOutput=0
  Zone2 : Outport  Port=2  InitialOutput=0
  Zone3 : Outport  Port=3  InitialOutput=0
  Starter : Outport  Port=4  InitialOutput=0
  ZoneR : Outport  Port=5  InitialOutput=0
  "R, X" : Outport  Port=6  InitialOutput=0
  wires:
  Voltage Current/2 -> Impedance Module/2
  Voltage Current/1 -> Impedance Module/1
  Impedance Module/1 -> Complex to Real-Imag/1
  Mux4/1 -> Zone4Z/1
  Mux3/1 -> Zone3Z/1
  Mux2/1 -> Zone2Z/1
  Mux1/1 -> Zone1Z/1
  <V/1 -> Zone R/2(<V), Zone 4/2(<V), Zone 3/2(<V), Zone 2/2(<V), Zone 1/2(<V)
  Complex to Real-Imag/2 -> Mux6/2, Mux/2
  Complex to Real-Imag/1 -> Mux6/1, Mux/1
  Zone 4/1(TRIP) -> Starter/1
  Zone 3/1(TRIP) -> Zone3/1
  Zone 2/1(TRIP) -> Zone2/1
  Zone 4/3(Zr) -> Mux4/2
  Zone 4/2(Zm) -> Mux4/1
  Zone 3/3(Zr) -> Mux3/2
  Zone 3/2(Zm) -> Mux3/1
  Zone 2/3(Zr) -> Mux2/2
  Zone 2/2(Zm) -> Mux2/1
  Zone 1/3(Zr) -> Mux1/2
  Zone 1/2(Zm) -> Mux1/1
  Zone 1/1(TRIP) -> Zone1/1
  Mux/1 -> Zone 2/1(Z), Zone R/1(Z), Zone 4/1(Z), Zone 3/1(Z), Zone 1/1(Z)
  C-G/1 -> Voltage Current/1
  Zone R/2(Zm) -> Mux5/1
  Zone R/3(Zr) -> Mux5/2
  Mux5/1 -> ZoneRZ/1
  Zone R/1(TRIP) -> ZoneR/1
  Mux6/1 -> "R, X"/1

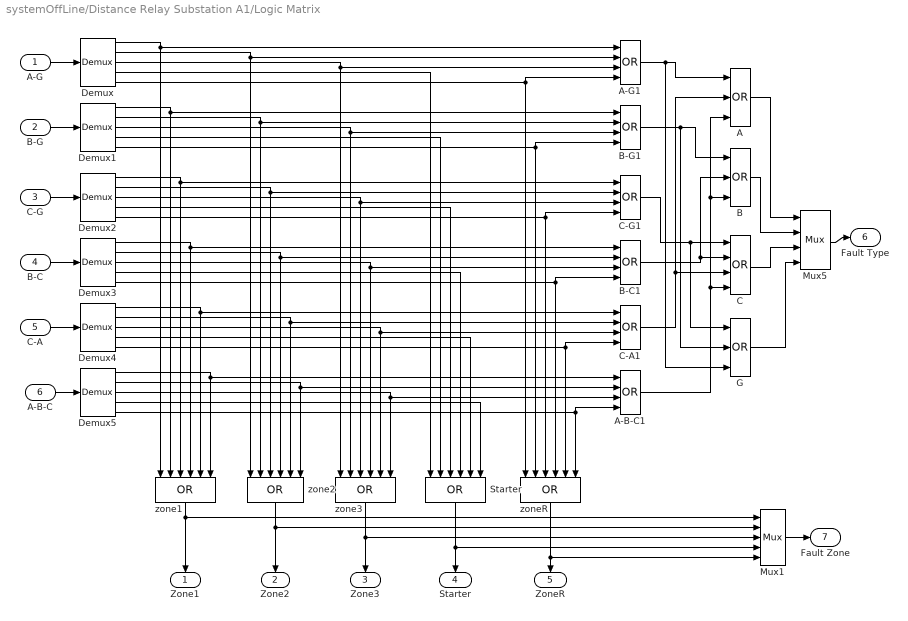
== system systemOffLine/Distance Relay Substation A1/Logic Matrix ==
  A-G : Inport
  B-G : Inport  Port=2
  C-G : Inport  Port=3
  B-C : Inport  Port=4
  C-A : Inport  Port=5
  A-B-C : Inport  Port=6
  A : Logic  Operator=OR  Inputs=3
  A-B-C1 : Logic  Operator=OR  Inputs=4
  "A-G1 " : Logic  Operator=OR  Inputs=4
  B : Logic  Operator=OR  Inputs=3
  B-C1 : Logic  Operator=OR  Inputs=4
  B-G1 : Logic  Operator=OR  Inputs=4
  C : Logic  Operator=OR  Inputs=4
  C-A1 : Logic  Operator=OR  Inputs=4
  C-G1 : Logic  Operator=OR  Inputs=4
  Demux{,1..5} (6 alike) : Demux  Outputs=5
  G : Logic  Operator=OR  Inputs=3
  Mux1 : Mux  Inputs=5
  Mux5 : Mux
  Starter : Logic  Operator=OR  Inputs=6
  zone1 : Logic  Operator=OR  Inputs=6
  zone2 : Logic  Operator=OR  Inputs=6
  zone3 : Logic  Operator=OR  Inputs=6
  zoneR : Logic  Operator=OR  Inputs=6
  " Zone1" : Outport  InitialOutput=0
  " Zone2" : Outport  Port=2  InitialOutput=0
  " Zone3" : Outport  Port=3  InitialOutput=0
  " Starter" : Outport  Port=4  InitialOutput=0
  " ZoneR" : Outport  Port=5  InitialOutput=0
  Fault Type : Outport  Port=6  InitialOutput=0
  Fault Zone : Outport  Port=7  InitialOutput=0
  wires:
  G/1 -> Mux5/4
  C/1 -> Mux5/3
  B/1 -> Mux5/2
  A/1 -> Mux5/1
  B-G1/1 -> G/2, B/1
  C-G1/1 -> G/1, C/1
  B-C1/1 -> C/2, B/2
  A-B-C1/1 -> B/3, A/3, C/4
  C-A1/1 -> A/2, C/3
  "A-G1 "/1 -> G/3, A/1
  A-G/1 -> Demux/1
  B-G/1 -> Demux1/1
  A-B-C/1 -> Demux5/1
  C-A/1 -> Demux4/1
  B-C/1 -> Demux3/1
  C-G/1 -> Demux2/1
  Mux5/1 -> Fault Type/1
  zone1/1 -> " Zone1"/1, Mux1/1
  zone2/1 -> Mux1/2, " Zone2"/1
  zoneR/1 -> Mux1/5, " ZoneR"/1
  zone3/1 -> " Zone3"/1, Mux1/3
  Starter/1 -> Mux1/4, " Starter"/1
  Mux1/1 -> Fault Zone/1
  Demux/5 -> zoneR/1, "A-G1 "/4
  Demux1/5 -> zoneR/2, B-G1/4
  Demux2/5 -> zoneR/3, C-G1/4
  Demux3/5 -> zoneR/4, B-C1/4
  Demux4/5 -> zoneR/5, C-A1/4
  Demux5/5 -> zoneR/6, A-B-C1/4
  Demux/1 -> "A-G1 "/1, zone1/1
  Demux1/1 -> B-G1/1, zone1/2
  Demux2/1 -> C-G1/1, zone1/3
  Demux3/1 -> B-C1/1, zone1/4
  Demux4/1 -> C-A1/1, zone1/5
  Demux5/1 -> A-B-C1/1, zone1/6
  Demux/2 -> "A-G1 "/2, zone2/1
  Demux1/2 -> B-G1/2, zone2/2
  Demux2/2 -> C-G1/2, zone2/3
  Demux3/2 -> B-C1/2, zone2/4
  Demux4/2 -> C-A1/2, zone2/5
  Demux5/2 -> A-B-C1/2, zone2/6
  Demux/3 -> "A-G1 "/3, zone3/1
  Demux1/3 -> B-G1/3, zone3/2
  Demux2/3 -> C-G1/3, zone3/3
  Demux3/3 -> B-C1/3, zone3/4
  Demux4/3 -> C-A1/3, zone3/5
  Demux5/3 -> A-B-C1/3, zone3/6
  Demux/4 -> Starter/1
  Demux1/4 -> Starter/2
  Demux2/4 -> Starter/3
  Demux3/4 -> Starter/4
  Demux4/4 -> Starter/5
  Demux5/4 -> Starter/6

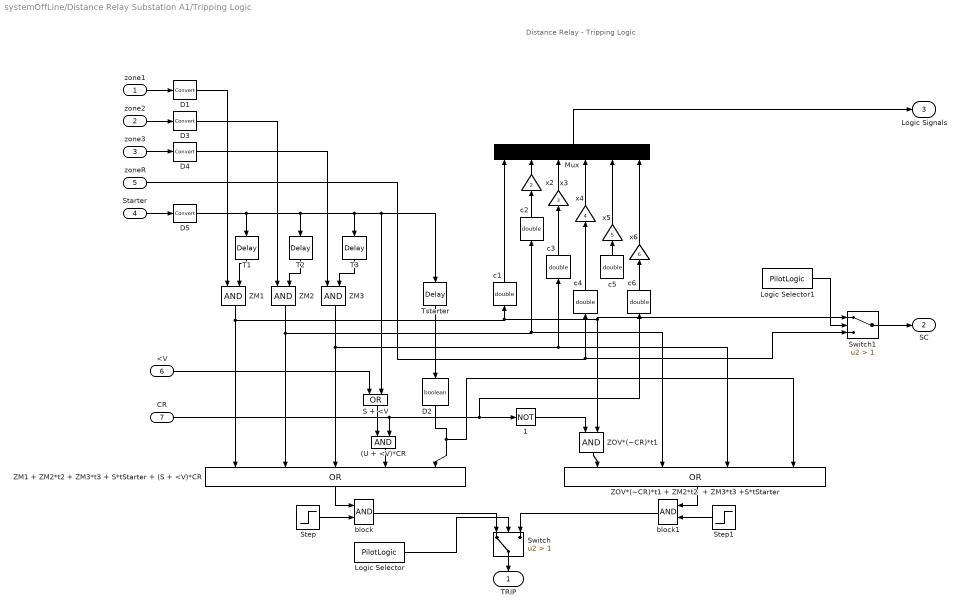
== system systemOffLine/Distance Relay Substation A1/Tripping Logic ==
  note: Distance Relay - Tripping Logic
  zone1 : Inport
  zone2 : Inport  Port=2
  zone3 : Inport  Port=3
  Starter : Inport  Port=4
  zoneR : Inport  Port=5
  <V : Inport  Port=6
  CR : Inport  Port=7
  (U + <V)*CR : Logic  AllPortsSameDT=off  OutDataTypeStr=boolean
  1 : Logic  Operator=NOT  AllPortsSameDT=off  OutDataTypeStr=boolean
  D{1,3..5} (4 alike) : DataTypeConversion
  D2 : DataTypeConversion  OutDataTypeStr=boolean
  Logic Selector : Constant  Value=PilotLogic  OutDataTypeStr=boolean
  Logic Selector1 : Constant  Value=PilotLogic  OutDataTypeStr=boolean
  Mux : Mux  Inputs=6
  S + <V : Logic  Operator=OR  AllPortsSameDT=off  OutDataTypeStr=boolean
  Step : Step  SampleTime=0
  Step1 : Step  SampleTime=0
  Switch : Switch  Criteria=u2 > Threshold  Threshold=1
  Switch1 : Switch  Criteria=u2 > Threshold  Threshold=1
  T1 : TransportDelay  DelayTime=ZoneTime(1)
  T2 : TransportDelay  DelayTime=ZoneTime(2)
  T3 : TransportDelay  DelayTime=ZoneTime(3)
  Tstarter : TransportDelay  DelayTime=Tstarter
  ZM1 : Logic  AllPortsSameDT=off  OutDataTypeStr=boolean
  ZM1 + ZM2*t2 + ZM3*t3 + S*tStarter + (S + <V)*CR : Logic  Operator=OR  Inputs=5
  ZM2 : Logic  AllPortsSameDT=off  OutDataTypeStr=boolean
  ZM3 : Logic  AllPortsSameDT=off  OutDataTypeStr=boolean
  ZOV*(~CR)*t1 : Logic  AllPortsSameDT=off  OutDataTypeStr=boolean
  ZOV*(~CR)*t1 + ZM2*t2  + ZM3*t3 +S*tStarter : Logic  Operator=OR  Inputs=4
  block : Logic  AllPortsSameDT=off  OutDataTypeStr=boolean
  block1 : Logic  AllPortsSameDT=off  OutDataTypeStr=boolean
  c{1..6} (6 alike) : DataTypeConversion  OutDataTypeStr=double
  x2 : Gain  Gain=2  SaturateOnIntegerOverflow=on  OutDataTypeStr=Inherit: Same as input  ParamDataTypeStr=Inherit: Same as input
  x3 : Gain  Gain=3  SaturateOnIntegerOverflow=on  OutDataTypeStr=Inherit: Same as input  ParamDataTypeStr=Inherit: Same as input
  x4 : Gain  Gain=4  SaturateOnIntegerOverflow=on  OutDataTypeStr=Inherit: Same as input  ParamDataTypeStr=Inherit: Same as input
  x5 : Gain  Gain=5  SaturateOnIntegerOverflow=on  OutDataTypeStr=Inherit: Same as input  ParamDataTypeStr=Inherit: Same as input
  x6 : Gain  Gain=6  SaturateOnIntegerOverflow=on  OutDataTypeStr=Inherit: Same as input  ParamDataTypeStr=Inherit: Same as input
  TRIP : Outport  InitialOutput=0
  SC : Outport  Port=2  InitialOutput=0
  Logic Signals : Outport  Port=3  InitialOutput=0
  wires:
  T1/1 -> ZM1/2
  T2/1 -> ZM2/2
  T3/1 -> ZM3/2
  ZM1/1 -> ZOV*(~CR)*t1/2, Switch1/1, c1/1, ZM1 + ZM2*t2 + ZM3*t3 + S*tStarter + (S + <V)*CR/1
  ZM2/1 -> c2/1, ZOV*(~CR)*t1 + ZM2*t2  + ZM3*t3 +S*tStarter/2, ZM1 + ZM2*t2 + ZM3*t3 + S*tStarter + (S + <V)*CR/2
  ZM3/1 -> c3/1, ZOV*(~CR)*t1 + ZM2*t2  + ZM3*t3 +S*tStarter/3, ZM1 + ZM2*t2 + ZM3*t3 + S*tStarter + (S + <V)*CR/3
  (U + <V)*CR/1 -> ZM1 + ZM2*t2 + ZM3*t3 + S*tStarter + (S + <V)*CR/4
  S + <V/1 -> (U + <V)*CR/1
  <V/1 -> S + <V/1
  x2/1 -> Mux/2
  x3/1 -> Mux/3
  x4/1 -> Mux/4
  x5/1 -> Mux/5
  x6/1 -> Mux/6
  Mux/1 -> Logic Signals/1
  ZOV*(~CR)*t1/1 -> ZOV*(~CR)*t1 + ZM2*t2  + ZM3*t3 +S*tStarter/1
  1/1 -> ZOV*(~CR)*t1/1
  ZM1 + ZM2*t2 + ZM3*t3 + S*tStarter + (S + <V)*CR/1 -> block/1
  Step/1 -> block/2
  Switch/1 -> TRIP/1
  Logic Selector/1 -> Switch/2
  block/1 -> Switch/1
  ZOV*(~CR)*t1 + ZM2*t2  + ZM3*t3 +S*tStarter/1 -> block1/1
  block1/1 -> Switch/3
  Step1/1 -> block1/2
  Switch1/1 -> SC/1
  Logic Selector1/1 -> Switch1/2
  zoneR/1 -> c4/1, Switch1/3
  c1/1 -> Mux/1
  c2/1 -> x2/1
  c3/1 -> x3/1
  c4/1 -> x4/1
  c5/1 -> x5/1
  c6/1 -> x6/1
  CR/1 -> 1/1, c6/1, (U + <V)*CR/2
  Tstarter/1 -> D2/1
  D2/1 -> ZOV*(~CR)*t1 + ZM2*t2  + ZM3*t3 +S*tStarter/4, ZM1 + ZM2*t2 + ZM3*t3 + S*tStarter + (S + <V)*CR/5
  zone1/1 -> D1/1
  D1/1 -> ZM1/1
  D3/1 -> ZM2/1
  zone2/1 -> D3/1
  zone3/1 -> D4/1
  D4/1 -> ZM3/1
  Starter/1 -> D5/1
  D5/1 -> T2/1, T3/1, Tstarter/1, S + <V/2, T1/1

== system systemOffLine/Distance Relay Substation A1/Undervoltage ==
  "Vabc  " : Inport
  Abs : Abs
  Abs1 : Abs
  Abs2 : Abs
  Demux2 : Demux  Outputs=3
  Logical Operator : Logic  Operator=OR  Inputs=3
  Relational Operator : RelationalOperator  Operator=<  InputSameDT=on
  Relational Operator1 : RelationalOperator  Operator=<  InputSameDT=on
  Relational Operator2 : RelationalOperator  Operator=<  InputSameDT=on
  underV  Threshold : Constant  Value=underV
  <V : Outport  InitialOutput=0
  wires:
  Demux2/3 -> Abs2/1
  Demux2/2 -> Abs1/1
  Abs1/1 -> Relational Operator2/1
  Abs2/1 -> Relational Operator1/1
  Demux2/1 -> Abs/1
  Abs/1 -> Relational Operator/1
  Relational Operator1/1 -> Logical Operator/3
  Relational Operator/1 -> Logical Operator/1
  Relational Operator2/1 -> Logical Operator/2
  Logical Operator/1 -> <V/1
  underV  Threshold/1 -> Relational Operator1/2, Relational Operator2/2, Relational Operator/2
  "Vabc  "/1 -> Demux2/1

== system systemOffLine/Distance Relay Substation A2/Analog filtering, signal  conditioning ==
  note: Acquisition Block- analog filtering,
      | signal conditioning, sampling.
  Vin : Inport
  Iin : Inport  Port=2
  CURRENTS : Subsystem
  Mux{1..4} (4 alike) : Mux  Inputs=3
  VOLTAGES : Subsystem
  Vf : Outport  InitialOutput=0
  If : Outport  Port=2  InitialOutput=0
  If0 : Outport  Port=3  InitialOutput=0
  vf : Outport  Port=4  InitialOutput=0
  if : Outport  Port=5  InitialOutput=0
  wires:
  CURRENTS/4(k0I0f) -> If0/1
  Mux4/1 -> if/1
  Mux3/1 -> If/1
  CURRENTS/7(icf) -> Mux4/3
  CURRENTS/6(ibf) -> Mux4/2
  CURRENTS/5(iaf) -> Mux4/1
  CURRENTS/3(ICf) -> Mux3/3
  CURRENTS/2(IBf) -> Mux3/2
  CURRENTS/1(IAf) -> Mux3/1
  Iin/1 -> CURRENTS/1(Iabc)
  Mux2/1 -> vf/1
  VOLTAGES/6(vcf) -> Mux2/3
  VOLTAGES/5(vbf) -> Mux2/2
  VOLTAGES/4(vaf) -> Mux2/1
  VOLTAGES/3(VCf) -> Mux1/3
  VOLTAGES/2(VBf) -> Mux1/2
  VOLTAGES/1(VAf) -> Mux1/1
  Vin/1 -> VOLTAGES/1(Vabc)
  Mux1/1 -> Vf/1

== system systemOffLine/Distance Relay Substation A2/Combination of Voltages  and Currents into 6 pairs  (for each type of fault) ==
  note: Voltage and current combination block
  Vf : Inport
  If : Inport  Port=2
  If0 : Inport  Port=3
  "Currents Ia, Ib, Ic, kIo" : Demux  Outputs=3
  Ia+kIo : Sum  SaturateOnIntegerOverflow=on  InputSameDT=on  OutDataTypeStr=Inherit: Same as first input
  Ia-Ib : Sum  Inputs=+-  SaturateOnIntegerOverflow=on  InputSameDT=on  OutDataTypeStr=Inherit: Same as first input
  Ib+kIo : Sum  SaturateOnIntegerOverflow=on  InputSameDT=on  OutDataTypeStr=Inherit: Same as first input
  Ib-Ic : Sum  Inputs=+-  SaturateOnIntegerOverflow=on  InputSameDT=on  OutDataTypeStr=Inherit: Same as first input
  Ic+kIo : Sum  SaturateOnIntegerOverflow=on  InputSameDT=on  OutDataTypeStr=Inherit: Same as first input
  Ic-Ia : Sum  Inputs=+-  SaturateOnIntegerOverflow=on  InputSameDT=on  OutDataTypeStr=Inherit: Same as first input
  Mux{10..15} (6 alike) : Mux  Inputs=2
  Va-Vb : Sum  Inputs=+-  SaturateOnIntegerOverflow=on  InputSameDT=on  OutDataTypeStr=Inherit: Same as first input
  Vb-Vc : Sum  Inputs=+-  SaturateOnIntegerOverflow=on  InputSameDT=on  OutDataTypeStr=Inherit: Same as first input
  Vc-Va : Sum  Inputs=+-  SaturateOnIntegerOverflow=on  InputSameDT=on  OutDataTypeStr=Inherit: Same as first input
  "Voltages Va,Vb, Vc" : Demux  Outputs=3
  "Volt, Curr A-G" : Outport  InitialOutput=0
  "Volt, Curr B-G" : Outport  Port=2  InitialOutput=0
  "Volt, Curr C-G" : Outport  Port=3  InitialOutput=0
  "Volt, Curr  B-C,B-C-G" : Outport  Port=4  InitialOutput=0
  "Volt, Curr C-A,C-A-G" : Outport  Port=5  InitialOutput=0
  "Volt, Curr A-B,A-B-C-G" : Outport  Port=6  InitialOutput=0
  wires:
  If0/1 -> Ib+kIo/2, Ia+kIo/2, Ic+kIo/2
  Mux13/1 -> "Volt, Curr  B-C,B-C-G"/1
  Vb-Vc/1 -> Mux13/1
  Ib-Ic/1 -> Mux13/2
  Mux12/1 -> "Volt, Curr C-G"/1
  Ic+kIo/1 -> Mux12/2
  If/1 -> "Currents Ia, Ib, Ic, kIo"/1
  "Voltages Va,Vb, Vc"/3 -> Vc-Va/1, Vb-Vc/2, Mux12/1
  "Voltages Va,Vb, Vc"/2 -> Vb-Vc/1, Mux11/1, Va-Vb/2
  "Voltages Va,Vb, Vc"/1 -> Va-Vb/1, Mux10/1, Vc-Va/2
  Vf/1 -> "Voltages Va,Vb, Vc"/1
  Mux15/1 -> "Volt, Curr A-B,A-B-C-G"/1
  Mux14/1 -> "Volt, Curr C-A,C-A-G"/1
  Vc-Va/1 -> Mux14/1
  Mux11/1 -> "Volt, Curr B-G"/1
  Mux10/1 -> "Volt, Curr A-G"/1
  Ia+kIo/1 -> Mux10/2
  Ib+kIo/1 -> Mux11/2
  Ic-Ia/1 -> Mux14/2
  Va-Vb/1 -> Mux15/1
  Ia-Ib/1 -> Mux15/2
  "Currents Ia, Ib, Ic, kIo"/2 -> Ia-Ib/2, Ib-Ic/1, Ib+kIo/1
  "Currents Ia, Ib, Ic, kIo"/3 -> Ic-Ia/1, Ib-Ic/2, Ic+kIo/1
  "Currents Ia, Ib, Ic, kIo"/1 -> Ia-Ib/1, Ic-Ia/2, Ia+kIo/1
